simulink model "PX30ees"  (R2015b)
settings: Solver=VariableStepAuto  StartTime=0.0  StopTime=3  RelTol=1e-3
settings Model: Creator=xmax1946  LastModifiedBy=xmax1946

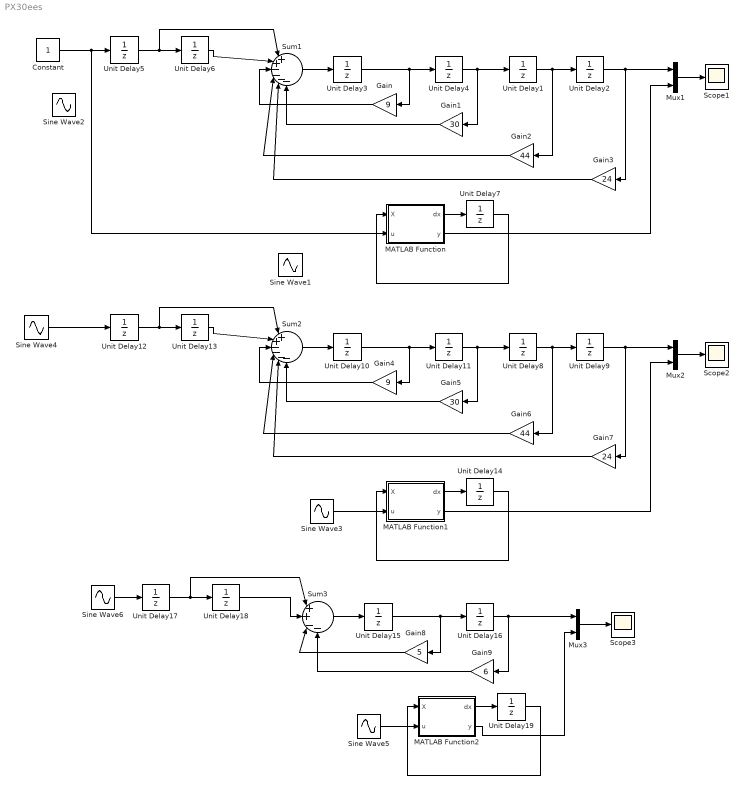
== system PX30ees ==
  Constant : Constant
  Gain : Gain  Gain=9
  Gain1 : Gain  Gain=30
  Gain2 : Gain  Gain=44
  Gain3 : Gain  Gain=24
  Gain4 : Gain  Gain=9
  Gain5 : Gain  Gain=30
  Gain6 : Gain  Gain=44
  Gain7 : Gain  Gain=24
  Gain8 : Gain  Gain=5
  Gain9 : Gain  Gain=6
  MATLAB Function : MATLAB Function  TreatAsAtomicUnit=on
  MATLAB Function1 : MATLAB Function  TreatAsAtomicUnit=on
  MATLAB Function2 : MATLAB Function  TreatAsAtomicUnit=on
  Mux1 : Mux  Inputs=2
  Mux2 : Mux  Inputs=2
  Mux3 : Mux  Inputs=2
  Scope1 : Scope
  Scope2 : Scope
  Scope3 : Scope
  Sine Wave1 : Sin  Samples=1  SampleTime=1
  Sine Wave2 : Sin  Phase=4  Samples=1  SampleTime=1
  Sine Wave3 : Sin  Samples=1  SampleTime=1
  Sine Wave4 : Sin  Phase=4  Samples=1  SampleTime=1
  Sine Wave5 : Sin  Samples=1  SampleTime=1
  Sine Wave6 : Sin  Phase=2  Samples=1  SampleTime=1
  Sum1 : Sum  Inputs=|++----
  Sum2 : Sum  Inputs=|++----
  Sum3 : Sum  Inputs=|++--
  Unit Delay{1,5..6,8,15} (5 alike) : UnitDelay  InitialCondition=1  SampleTime=-1
  Unit Delay{2..4,9..11,16} (7 alike) : UnitDelay  InitialCondition=2  SampleTime=-1
  Unit Delay12 : UnitDelay  InitialCondition=sin(3)  SampleTime=-1
  Unit Delay13 : UnitDelay  InitialCondition=sin(2)  SampleTime=-1
  Unit Delay14 : UnitDelay  InitialCondition=[-49.2826;-32.5057;-13.9830;-2.3763]  SampleTime=-1
  Unit Delay17 : UnitDelay  InitialCondition=sin(1)  SampleTime=-1
  Unit Delay18 : UnitDelay  InitialCondition=sin(0)  SampleTime=-1
  Unit Delay19 : UnitDelay  InitialCondition=[-7;-2.5]  SampleTime=-1
  Unit Delay7 : UnitDelay  InitialCondition=[-49.1250;-32.25;-13.5;-2.0556]  SampleTime=-1
  wires:
  Mux1/1 -> Scope1/1
  Unit Delay3/1 -> Unit Delay4/1, Gain/1
  Sum1/1 -> Unit Delay3/1
  Gain/1 -> Sum1/3
  Unit Delay4/1 -> Gain1/1, Unit Delay1/1
  Unit Delay1/1 -> Gain2/1, Unit Delay2/1
  Unit Delay2/1 -> Gain3/1, Mux1/1
  Gain2/1 -> Sum1/4
  Gain3/1 -> Sum1/5
  Gain1/1 -> Sum1/6
  Unit Delay5/1 -> Sum1/1, Unit Delay6/1
  Unit Delay6/1 -> Sum1/2
  MATLAB Function/1(dx) -> Unit Delay7/1
  Unit Delay7/1 -> MATLAB Function/1(X)
  MATLAB Function/2(y) -> Mux1/2
  Constant/1 -> MATLAB Function/2(u), Unit Delay5/1
  Mux2/1 -> Scope2/1
  Unit Delay10/1 -> Unit Delay11/1, Gain4/1
  Sum2/1 -> Unit Delay10/1
  Gain4/1 -> Sum2/3
  Unit Delay11/1 -> Gain5/1, Unit Delay8/1
  Unit Delay8/1 -> Gain6/1, Unit Delay9/1
  Unit Delay9/1 -> Gain7/1, Mux2/1
  Gain6/1 -> Sum2/4
  Gain7/1 -> Sum2/5
  Gain5/1 -> Sum2/6
  Unit Delay12/1 -> Sum2/1, Unit Delay13/1
  Unit Delay13/1 -> Sum2/2
  MATLAB Function1/1(dx) -> Unit Delay14/1
  Unit Delay14/1 -> MATLAB Function1/1(X)
  MATLAB Function1/2(y) -> Mux2/2
  Sine Wave4/1 -> Unit Delay12/1
  Sine Wave3/1 -> MATLAB Function1/2(u)
  Mux3/1 -> Scope3/1
  Unit Delay15/1 -> Unit Delay16/1, Gain8/1
  Sum3/1 -> Unit Delay15/1
  Gain8/1 -> Sum3/3
  Unit Delay16/1 -> Mux3/1, Gain9/1
  Unit Delay17/1 -> Sum3/1, Unit Delay18/1
  Unit Delay18/1 -> Sum3/2
  MATLAB Function2/1(dx) -> Unit Delay19/1
  Unit Delay19/1 -> MATLAB Function2/1(X)
  MATLAB Function2/2(y) -> Mux3/2
  Gain9/1 -> Sum3/4
  Sine Wave6/1 -> Unit Delay17/1
  Sine Wave5/1 -> MATLAB Function2/2(u)

== matlab function PX30ees/MATLAB Function1 ==
  data: X input; dx output; u input; y output
function [dx,y]= fcn(X,u)

A=[-2,1,0,0
   0,-2,1,0
   0,0,-2,0
   0,0,0,-3];
B=[0;0;1;1];
C=[-4,12,-17,18];

dx=A*X+B*u;
y=C*X;

% [-0.0379;1.9455;-4.5769;6.5769]
% [-8.8993;-6.1657,-1.8636,.4839]
% [-4.231;-2.7423;-.7343;.3056]
% [-37.9663;-24.1346;-9.4423;-1.1538]
%   [-27.3125;-16.3864;-5.5682;-0.2929]
% [-27.5625;-16.5682;-5.6591;-0.3131]
% [-49.1250;-32.25;-13.5;-2.0556]
% [-49.2826;-32.5057;-13.9830;-2.3763]

== matlab function PX30ees/MATLAB Function ==
  data: X input; dx output; u input; y output
function [dx,y]= fcn(X,u)

A=[-2,1,0,0
   0,-2,1,0
   0,0,-2,0
   0,0,0,-3];
B=[0;0;1;1];
C=[-4,12,-17,18];

dx=A*X+B*u;
y=C*X;

% [-0.0379;1.9455;-4.5769;6.5769]
% [-8.8993;-6.1657,-1.8636,.4839]
% [-4.231;-2.7423;-.7343;.3056]
% [-37.9663;-24.1346;-9.4423;-1.1538]
%   [-27.3125;-16.3864;-5.5682;-0.2929]
% [-27.5625;-16.5682;-5.6591;-0.3131]
% [-49.1250;-32.25;-13.5;-2.0556]
% [-49.2826;-32.5057;-13.9830;-2.3763]

== matlab function PX30ees/MATLAB Function2 ==
  data: X input; dx output; u input; y output
function [dx,y]= fcn(X,u)

A=[-2,0;0,-3];
B=[1;1];
C=[-1,2];

dx=A*X+B*u;
y=C*X;
% [-6,-2];
% [-7,-2,5]
